simulink library "Solver_DS_SF"  (Simulink 7.1)
libraries: simulink x65
(part 1 of 2)
settings Model: Creator=Jin  LastModifiedBy=Jin

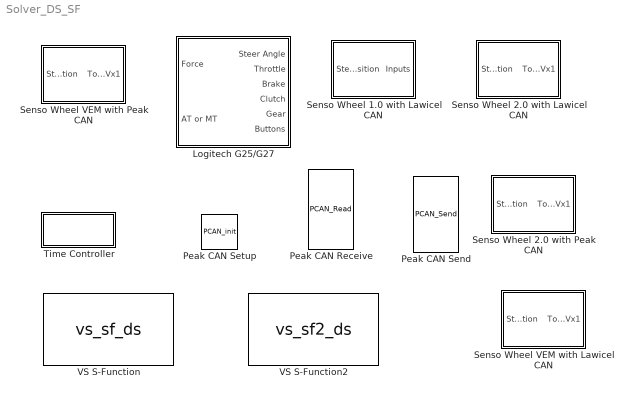
== system Solver_DS_SF ==
  Logitech G25/G27 : Subsystem
      mask Type: CarSim DS
      mask Description:
      | Logitech G25 Steering Wheel for CarSim/TruckSim Driving Simulator
      | 
      | Input 1: Force feedback
      | Input 2: AT mode (1), MT mode (-1)
      | 
      | Output 1: Steering Angle (-450deg - 450deg)
      | Output 2: Throttle position (0-1)
      | Output 3: Brake position (0-1)
      | Output 4: Clutch position (0-1)
      | Output 5: Gear shift
      |                 MT Mode:
      |                                 -1:  R
      |                               1-6: Gear 1-6
      |                 AT Mode:
      |                               button 1: Down shift
      |                               button 2: Upshift
      | Output 6: Other 14 buttons.
      mask Display: image(imread('G25.jpg'))
  Peak CAN Receive : S-Function  FunctionName=PCAN_Read  Parameters=id,TimeStep,nOut,bits_define  EnableBusSupport=off  mask{id=529, TimeStep=0.01, bits_define={[0:31],[32:47],[48:63]}, portnames={'Position','Speed','Motor Torque'}}
      mask prompts: id "CAN ID"; TimeStep "Sample time"; bits_define "Bit defination (cell array):"; portnames "Port name (cell array):"
      mask help: Peak-System USB CAN Receive.
      mask init:
      | %set_param(gcb, 'InitFcn', ['CAN_h=' adapter '_handle;']);
      | nOut=length(bits_define);
      | [bits_define]=formatbit(bits_define,portnames,1);
      | set_param(gcb, 'Parameters', ['id,TimeStep,nOut,bits_define']);
      mask Display: port_label('output',1,'Position ');port_label('output',2,'Speed ');port_label('output',3,'Motor Torque ');
  Peak CAN Send : S-Function  FunctionName=PCAN_Send  Parameters=id,len,TimeStep,nOut,bits_define  EnableBusSupport=off  mask{id=513, len=8, TimeStep=0.02, bits_define={[0:15],[16:31],[32:47],[48:63]}, portnames={'Torque Set Value','Friction','Damping','Spring Stiffness'}}
      mask prompts: id "CAN ID"; len "Data Length"; TimeStep "Sample time"; bits_define "Bit defination (cell array):"; portnames "Port name (cell array):"
      mask help: Peak-System USB CAN send
      mask init:
      | nOut=length(bits_define);
      | [bits_define]=formatbit(bits_define,portnames,0);
      | set_param(gcb, 'Parameters', ['id,len,TimeStep,nOut,bits_define']);
      mask StyleString: edit,popup(1|2|3|4|5|6|7|8),edit,edit,edit
      mask Display: port_label('input',1,' Torque Set Value');port_label('input',2,' Friction');port_label('input',3,' Damping');port_label('input',4,' Spring Stiffness');
  Peak CAN Setup : S-Function  Priority=1  FunctionName=PCAN_init  Parameters=CAN_MODE,szBitrate  EnableBusSupport=off  mask{CAN_MODE=Standard (11-bit), szBitrate=1000}
      mask prompts: CAN_MODE "CAN identifier range:"; szBitrate "Baud rate (kbps):"
      mask help: Peak-System USB CAN setup
      mask StyleString: popup(Standard (11-bit)|Extended (29-bit)),popup(1000|500|250|100|50|20|10|5)
      mask Display: image(imread('Peak_CAN.jpg'));
  Senso Wheel 1.0 with Lawicel CAN : Subsystem  Orientation=left  Priority=3
      mask Display: image(imread('SensoDrive.jpg'))
  Senso Wheel 2.0 with Lawicel CAN : Subsystem  Orientation=left  Priority=3
      mask Display: image(imread('SensoDrive.jpg'))
  Senso Wheel 2.0 with Peak CAN : Subsystem  Orientation=left  Priority=3
      mask Display: image(imread('SensoDrive.jpg'))
  Senso Wheel VEM with Lawicel CAN : Subsystem  Orientation=left  Priority=3
      mask Display: image(imread('SensoDrive.jpg'))
  Senso Wheel VEM with Peak CAN : Subsystem  Orientation=left  Priority=3  AncestorBlock=Solver_DS_SF/Senso Wheel 2.0 with Peak CAN
      mask Display: image(imread('SensoDrive.jpg'))
  Time Controller : Subsystem  AncestorBlock=Solver_SF/Time Controller  mask(CarSim DS){}
      mask help: This Real-Time control block enables the Simulink system running at real time mode.
      mask init:
      | TimeStep=str2num(get_param(gcs,'FixedStep'));
      mask Display: disp('RT Enable');
  VS S-Function : S-Function  Priority=1  FunctionName=vs_sf_ds  Parameters='simfile.sim'  EnableBusSupport=off  mask(Vehicle math model library){SIMFILE=simfile.sim}
      mask prompts: SIMFILE "Simfile name:"
      mask help:
      | The vehicle code on this S-Function determine which solver is used for vehicle type that is simulated.
      |
      | Simfile lists the names of the main files that will be read and written by the solver program.
      mask init:
      | set_param(gcb, 'Parameters', ['''',SIMFILE,'''']);
      mask Display: image(imread('car_ds.bmp'))
  VS S-Function2 : S-Function  Priority=1  FunctionName=vs_sf2_ds  Parameters='simfile.sim'  EnableBusSupport=off  mask(Vehicle math model library){SIMFILE=simfile.sim}
      mask prompts: SIMFILE "Simfile name:"
      mask help:
      | The vehicle code on this S-Function determine which solver is used for vehicle type that is simulated.
      |
      | Simfile lists the names of the main files that will be read and written by the solver program.
      mask init:
      | set_param(gcb, 'Parameters', ['''',SIMFILE,'''']);
      mask Display: image(imread('car_ds2.bmp'))

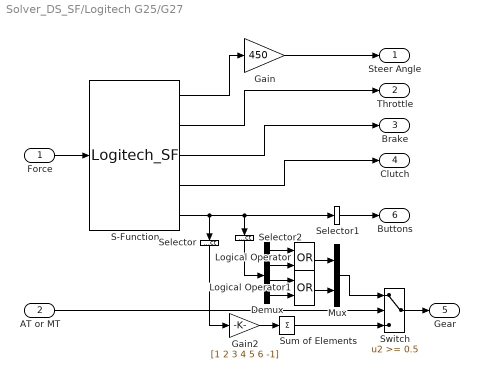
== system Solver_DS_SF/Logitech G25/G27 ==
  Force : Inport
  AT or MT : Inport  Port=2
  Demux : Demux
  Gain : Gain  Gain=450
  Gain2 : Gain  Gain=[1 2 3 4 5 6 -1]
  Logical Operator : Logic  Operator=OR  AllPortsSameDT=off  OutDataTypeStr=boolean  OutDataTypeMode=boolean
  Logical Operator1 : Logic  Operator=OR  AllPortsSameDT=off  OutDataTypeStr=boolean  OutDataTypeMode=boolean
  Mux : Mux  Inputs=2
  S-Function : S-Function  FunctionName=Logitech_SF  Parameters=19  EnableBusSupport=off
  Selector : Selector  Orientation=down  IndexOptions=Index vector (dialog)  Indices=[9 10 11 12 13 14 15]  OutputSizes=1
  Selector1 : Selector  IndexOptions=Index vector (dialog)  Indices=[1 2 3 4 5 6 7 8 16 17 18 19]  OutputSizes=1
  Selector2 : Selector  Orientation=down  IndexOptions=Index vector (dialog)  Indices=[9 6 10 5]  OutputSizes=1
  Sum of Elements : Sum  Inputs=+
  Switch : Switch  Threshold=0.5
  Steer Angle : Outport
  Throttle : Outport  Port=2
  Brake : Outport  Port=3
  Clutch : Outport  Port=4
  Gear : Outport  Port=5
  Buttons : Outport  Port=6
  wires:
  Mux/1 -> Switch/1
  Logical Operator1/1 -> Mux/2
  Logical Operator/1 -> Mux/1
  Demux/4 -> Logical Operator1/2
  Demux/3 -> Logical Operator1/1
  Demux/2 -> Logical Operator/2
  Demux/1 -> Logical Operator/1
  Selector2/1 -> Demux/1
  S-Function/1 -> Gain/1
  S-Function/2 -> Throttle/1
  Force/1 -> S-Function/1
  S-Function/3 -> Brake/1
  S-Function/4 -> Clutch/1
  S-Function/5 -> Selector2/1, Selector1/1, Selector/1
  Gain/1 -> Steer Angle/1
  Gain2/1 -> Sum of Elements/1
  Selector1/1 -> Buttons/1
  Selector/1 -> Gain2/1
  Sum of Elements/1 -> Switch/3
  AT or MT/1 -> Switch/2
  Switch/1 -> Gear/1

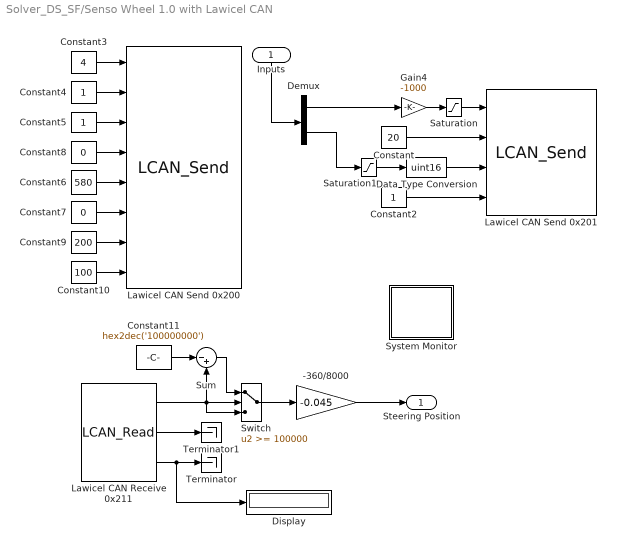
== system Solver_DS_SF/Senso Wheel 1.0 with Lawicel CAN ==
  Inputs : Inport  Orientation=down
  -360/8000 : Gain  Gain=-0.045  SaturateOnIntegerOverflow=on  OutDataTypeStr=Inherit: Same as input  ParamDataTypeStr=Inherit: Same as input
  Constant : Constant  Value=20  OutDataTypeStr=uint16  OutDataTypeMode=uint16
  Constant10 : Constant  Value=100  OutDataTypeStr=uint8  OutDataTypeMode=uint8
  Constant11 : Constant  Value=hex2dec('100000000')  VectorParams1D=off
  Constant2 : Constant  OutDataTypeStr=uint16  OutDataTypeMode=uint16
  Constant3 : Constant  Value=4  OutDataTypeStr=uint8  OutDataTypeMode=uint8
  Constant4 : Constant  OutDataTypeStr=uint8  OutDataTypeMode=uint8
  Constant5 : Constant  OutDataTypeStr=uint8  OutDataTypeMode=uint8
  Constant6 : Constant  Value=580  OutDataTypeStr=uint16  OutDataTypeMode=uint16
  Constant7 : Constant  Value=0  OutDataTypeStr=int16  OutDataTypeMode=int16
  Constant8 : Constant  Value=0  OutDataTypeStr=uint8  OutDataTypeMode=uint8
  Constant9 : Constant  Value=200  OutDataTypeStr=uint8  OutDataTypeMode=uint8
  Data Type Conversion : DataTypeConversion  OutDataTypeStr=uint16  OutDataTypeMode=uint16  RndMeth=Zero
  Demux : Demux  Outputs=2
  Display : Display
  Gain4 : Gain  Gain=-1000  SaturateOnIntegerOverflow=on  OutDataTypeStr=Inherit: Same as input  ParamDataTypeStr=Inherit: Same as input
  Lawicel CAN Receive 0x211 : S-Function  FunctionName=LCAN_Read  Parameters=1,CAN_MODE,id,TimeStep,nOut,bits_define  EnableBusSupport=off  mask{adapter=CAN1, CAN_MODE=Standard (11-bit), id=529, TimeStep=0.010, bits_define={[0:31],[32:47],[48:63]}, portnames={'Position','Speed','Motor Torque'}}
      mask prompts: adapter "CAN adapter"; CAN_MODE "CAN identifier range:"; id "CAN ID"; TimeStep "Sample time"; bits_define "Bit defination (cell array):"; portnames "Port name (cell array):"
      mask init:
      | nOut=length(bits_define);
      | [bits_define]=formatbit(bits_define,portnames,1);
      | set_param(gcb, 'Parameters', [adapter(4) ',CAN_MODE,id,TimeStep,nOut,bits_define']);
      mask StyleString: popup(CAN1|CAN2|CAN3|CAN4),popup(Standard (11-bit)|Extended (29-bit)),edit,edit,edit,edit
      mask Display: port_label('output',1,'Position ');port_label('output',2,'Speed ');port_label('output',3,'Motor Torque ');
  Lawicel CAN Send 0x200 : S-Function  FunctionName=LCAN_Send  Parameters=1,CAN_MODE,id,len,TimeStep,nOut,bits_define  EnableBusSupport=off  mask{adapter=CAN1, CAN_MODE=Standard (11-bit), id=512, len=8, TimeStep=0.025, bits_define={[0:3],[4:7],[8:11],[12:15],[16:31],[32:47],[48:55],[56:63]}, portnames={'Control Word','Operating Mode','Watch Dog','Position Limit','End Stop Position','Position Offset','Set Torque Limit','Peak Torque Limit'}}
      mask prompts: adapter "CAN adapter"; CAN_MODE "CAN identifier range:"; id "CAN ID"; len "Data Length"; TimeStep "Sample time"; bits_define "Bit defination (cell array):"; portnames "Port name (cell array):"
      mask init:
      | nOut=length(bits_define);
      | [bits_define]=formatbit(bits_define,portnames,0);
      | set_param(gcb, 'Parameters', [adapter(4) ',CAN_MODE,id,len,TimeStep,nOut,bits_define']);
      mask StyleString: popup(CAN1|CAN2|CAN3|CAN4),popup(Standard (11-bit)|Extended (29-bit)),edit,popup(1|2|3|4|5|6|7|8),edit,edit,edit
      mask Display: port_label('input',1,' Control Word');port_label('input',2,' Operating Mode');port_label('input',3,' Watch Dog');port_label('input',4,' Position Limit');port_label('input',5,' End Stop Position');port_label('input',6,' Position Offset');port_label('input',7,' Set Torque Limit');port_label('input',8,' Peak Torque Limit');
  Lawicel CAN Send 0x201 : S-Function  FunctionName=LCAN_Send  Parameters=1,CAN_MODE,id,len,TimeStep,nOut,bits_define  EnableBusSupport=off  mask{adapter=CAN1, CAN_MODE=Standard (11-bit), id=513, len=8, TimeStep=0.02, bits_define={[0:15],[16:31],[32:47],[48:63]}, portnames={'Torque Set Value','Friction','Damping','Spring Stiffness'}}
      mask prompts: adapter "CAN adapter"; CAN_MODE "CAN identifier range:"; id "CAN ID"; len "Data Length"; TimeStep "Sample time"; bits_define "Bit defination (cell array):"; portnames "Port name (cell array):"
      mask init:
      | nOut=length(bits_define);
      | [bits_define]=formatbit(bits_define,portnames,0);
      | set_param(gcb, 'Parameters', [adapter(4) ',CAN_MODE,id,len,TimeStep,nOut,bits_define']);
      mask StyleString: popup(CAN1|CAN2|CAN3|CAN4),popup(Standard (11-bit)|Extended (29-bit)),edit,popup(1|2|3|4|5|6|7|8),edit,edit,edit
      mask Display: port_label('input',1,' Torque Set Value');port_label('input',2,' Friction');port_label('input',3,' Damping');port_label('input',4,' Spring Stiffness');
  Saturation : Saturate  UpperLimit=14500  LowerLimit=-14500
  Saturation1 : Saturate  UpperLimit=200  LowerLimit=40
  Sum : Sum  Inputs=|-+  SaturateOnIntegerOverflow=on
  Switch : Switch  Threshold=100000  SaturateOnIntegerOverflow=on
  System Monitor : Subsystem
  Terminator : Terminator
  Terminator1 : Terminator
  Steering Position : Outport
  wires:
  Constant/1 -> Lawicel CAN Send 0x201/2
  Constant2/1 -> Lawicel CAN Send 0x201/4
  Constant3/1 -> Lawicel CAN Send 0x200/1
  Constant4/1 -> Lawicel CAN Send 0x200/2
  Constant5/1 -> Lawicel CAN Send 0x200/3
  Constant8/1 -> Lawicel CAN Send 0x200/4
  Constant6/1 -> Lawicel CAN Send 0x200/5
  Constant7/1 -> Lawicel CAN Send 0x200/6
  Constant9/1 -> Lawicel CAN Send 0x200/7
  Constant10/1 -> Lawicel CAN Send 0x200/8
  Lawicel CAN Receive 0x211/2 -> Terminator1/1
  Lawicel CAN Receive 0x211/3 -> Terminator/1, Display/1
  Lawicel CAN Receive 0x211/1 -> Sum/2, Switch/2, Switch/3
  -360/8000/1 -> Steering Position/1
  Gain4/1 -> Saturation/1
  Saturation/1 -> Lawicel CAN Send 0x201/1
  Constant11/1 -> Sum/1
  Sum/1 -> Switch/1
  Switch/1 -> -360/8000/1
  Inputs/1 -> Demux/1
  Demux/1 -> Gain4/1
  Demux/2 -> Saturation1/1
  Saturation1/1 -> Data Type Conversion/1
  Data Type Conversion/1 -> Lawicel CAN Send 0x201/3

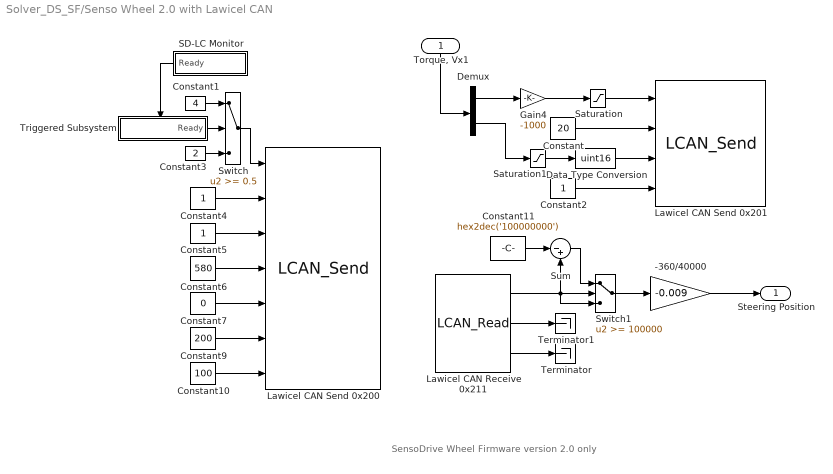
== system Solver_DS_SF/Senso Wheel 2.0 with Lawicel CAN ==
  note: SensoDrive Wheel Firmware version 2.0 only
  "Torque, Vx1" : Inport  Orientation=down
  -360/40000 : Gain  Gain=-0.009  SaturateOnIntegerOverflow=on  OutDataTypeStr=Inherit: Same as input  ParamDataTypeStr=Inherit: Same as input
  Constant : Constant  Value=20  OutDataTypeStr=uint16  OutDataTypeMode=uint16
  Constant1 : Constant  Value=4  OutDataTypeStr=uint8  OutDataTypeMode=uint8
  Constant10 : Constant  Value=100  OutDataTypeStr=uint8  OutDataTypeMode=uint8
  Constant11 : Constant  Value=hex2dec('100000000')  VectorParams1D=off
  Constant2 : Constant  OutDataTypeStr=uint16  OutDataTypeMode=uint16
  Constant3 : Constant  Value=2  OutDataTypeStr=uint8  OutDataTypeMode=uint8
  Constant4 : Constant  OutDataTypeStr=uint8  OutDataTypeMode=uint8
  Constant5 : Constant  OutDataTypeStr=uint8  OutDataTypeMode=uint8
  Constant6 : Constant  Value=580  OutDataTypeStr=uint16  OutDataTypeMode=uint16
  Constant7 : Constant  Value=0  OutDataTypeStr=int16  OutDataTypeMode=int16
  Constant9 : Constant  Value=200  OutDataTypeStr=uint8  OutDataTypeMode=uint8
  Data Type Conversion : DataTypeConversion  OutDataTypeStr=uint16  OutDataTypeMode=uint16  RndMeth=Zero
  Demux : Demux  Outputs=2
  Gain4 : Gain  Gain=-1000  SaturateOnIntegerOverflow=on  OutDataTypeStr=Inherit: Same as input  ParamDataTypeStr=Inherit: Same as input
  Lawicel CAN Receive 0x211 : S-Function  FunctionName=LCAN_Read  Parameters=1,CAN_MODE,id,TimeStep,nOut,bits_define  EnableBusSupport=off  mask{adapter=CAN1, CAN_MODE=Standard (11-bit), id=529, TimeStep=0.010, bits_define={[0:31],[32:47],[48:63]}, portnames={'Position','Speed','Motor Torque'}}
      mask prompts: adapter "CAN adapter"; CAN_MODE "CAN identifier range:"; id "CAN ID"; TimeStep "Sample time"; bits_define "Bit defination (cell array):"; portnames "Port name (cell array):"
      mask init:
      | nOut=length(bits_define);
      | [bits_define]=formatbit(bits_define,portnames,1);
      | set_param(gcb, 'Parameters', [adapter(4) ',CAN_MODE,id,TimeStep,nOut,bits_define']);
      mask StyleString: popup(CAN1|CAN2|CAN3|CAN4),popup(Standard (11-bit)|Extended (29-bit)),edit,edit,edit,edit
      mask Display: port_label('output',1,'Position ');port_label('output',2,'Speed ');port_label('output',3,'Motor Torque ');
  Lawicel CAN Send 0x200 : S-Function  Priority=3  FunctionName=LCAN_Send  Parameters=1,CAN_MODE,id,len,TimeStep,nOut,bits_define  EnableBusSupport=off  mask{adapter=CAN1, CAN_MODE=Standard (11-bit), id=512, len=8, TimeStep=0.025, bits_define={[0:3],[4:7],[8:15],[16:31],[32:47],[48:55],[56:63]}, portnames={'Control Word','Operating Mode','Aux. Functions','End Stop Position','Position Offset','Set Torque Limit','Peak Torque Limit'}}
      mask prompts: adapter "CAN adapter"; CAN_MODE "CAN identifier range:"; id "CAN ID"; len "Data Length"; TimeStep "Sample time"; bits_define "Bit defination (cell array):"; portnames "Port name (cell array):"
      mask init:
      | nOut=length(bits_define);
      | [bits_define]=formatbit(bits_define,portnames,0);
      | set_param(gcb, 'Parameters', [adapter(4) ',CAN_MODE,id,len,TimeStep,nOut,bits_define']);
      mask StyleString: popup(CAN1|CAN2|CAN3|CAN4),popup(Standard (11-bit)|Extended (29-bit)),edit,popup(1|2|3|4|5|6|7|8),edit,edit,edit
      mask Display: port_label('input',1,' Control Word');port_label('input',2,' Operating Mode');port_label('input',3,' Aux. Functions');port_label('input',4,' End Stop Position');port_label('input',5,' Position Offset');port_label('input',6,' Set Torque Limit');port_label('input',7,' Peak Torque Limit');
  Lawicel CAN Send 0x201 : S-Function  FunctionName=LCAN_Send  Parameters=1,CAN_MODE,id,len,TimeStep,nOut,bits_define  EnableBusSupport=off  mask{adapter=CAN1, CAN_MODE=Standard (11-bit), id=513, len=8, TimeStep=0.02, bits_define={[0:15],[16:31],[32:47],[48:63]}, portnames={'Torque Set Value','Friction','Damping','Spring Stiffness'}}
      mask prompts: adapter "CAN adapter"; CAN_MODE "CAN identifier range:"; id "CAN ID"; len "Data Length"; TimeStep "Sample time"; bits_define "Bit defination (cell array):"; portnames "Port name (cell array):"
      mask init:
      | nOut=length(bits_define);
      | [bits_define]=formatbit(bits_define,portnames,0);
      | set_param(gcb, 'Parameters', [adapter(4) ',CAN_MODE,id,len,TimeStep,nOut,bits_define']);
      mask StyleString: popup(CAN1|CAN2|CAN3|CAN4),popup(Standard (11-bit)|Extended (29-bit)),edit,popup(1|2|3|4|5|6|7|8),edit,edit,edit
      mask Display: port_label('input',1,' Torque Set Value');port_label('input',2,' Friction');port_label('input',3,' Damping');port_label('input',4,' Spring Stiffness');
  SD-LC Monitor : Subsystem  Orientation=left  Priority=4
  Saturation : Saturate  UpperLimit=14500  LowerLimit=-14500
  Saturation1 : Saturate  UpperLimit=200  LowerLimit=40
  Sum : Sum  Inputs=|-+  SaturateOnIntegerOverflow=on
  Switch : Switch  Threshold=0.5  SaturateOnIntegerOverflow=on
  Switch1 : Switch  Threshold=100000  SaturateOnIntegerOverflow=on
  Terminator : Terminator
  Terminator1 : Terminator
  Triggered Subsystem : Subsystem  TreatAsAtomicUnit=on
  Steering Position : Outport
  wires:
  Switch1/1 -> -360/40000/1
  Sum/1 -> Switch1/1
  Constant11/1 -> Sum/1
  -360/40000/1 -> Steering Position/1
  Lawicel CAN Receive 0x211/1 -> Sum/2, Switch1/2, Switch1/3
  Lawicel CAN Receive 0x211/3 -> Terminator/1
  Lawicel CAN Receive 0x211/2 -> Terminator1/1
  Data Type Conversion/1 -> Lawicel CAN Send 0x201/3
  Saturation1/1 -> Data Type Conversion/1
  Demux/2 -> Saturation1/1
  Demux/1 -> Gain4/1
  "Torque, Vx1"/1 -> Demux/1
  Saturation/1 -> Lawicel CAN Send 0x201/1
  Gain4/1 -> Saturation/1
  Constant2/1 -> Lawicel CAN Send 0x201/4
  Constant/1 -> Lawicel CAN Send 0x201/2
  Triggered Subsystem/1(Ready) -> Switch/2
  Constant1/1 -> Switch/1
  Constant3/1 -> Switch/3
  Switch/1 -> Lawicel CAN Send 0x200/1
  SD-LC Monitor/1(Ready) -> Triggered Subsystem/Trigger
  Constant10/1 -> Lawicel CAN Send 0x200/7
  Constant9/1 -> Lawicel CAN Send 0x200/6
  Constant7/1 -> Lawicel CAN Send 0x200/5
  Constant6/1 -> Lawicel CAN Send 0x200/4
  Constant5/1 -> Lawicel CAN Send 0x200/3
  Constant4/1 -> Lawicel CAN Send 0x200/2

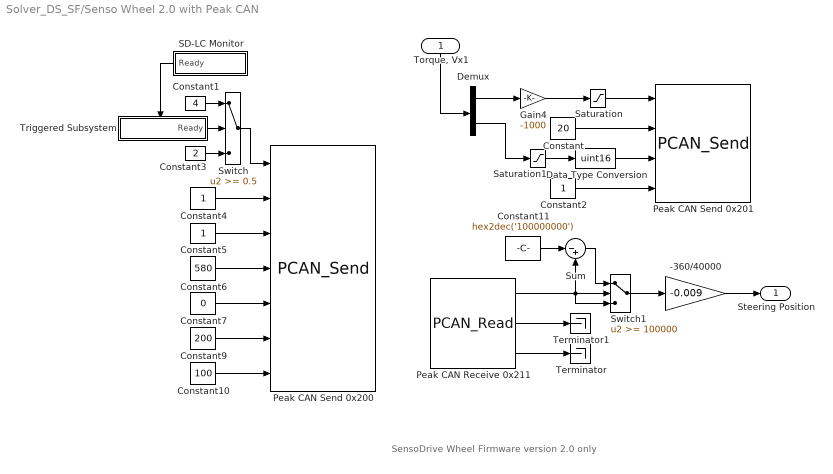
== system Solver_DS_SF/Senso Wheel 2.0 with Peak CAN ==
  note: SensoDrive Wheel Firmware version 2.0 only
  "Torque, Vx1" : Inport  Orientation=down
  -360/40000 : Gain  Gain=-0.009  SaturateOnIntegerOverflow=on  OutDataTypeStr=Inherit: Same as input  ParamDataTypeStr=Inherit: Same as input
  Constant : Constant  Value=20  OutDataTypeStr=uint16  OutDataTypeMode=uint16
  Constant1 : Constant  Value=4  OutDataTypeStr=uint8  OutDataTypeMode=uint8
  Constant10 : Constant  Value=100  OutDataTypeStr=uint8  OutDataTypeMode=uint8
  Constant11 : Constant  Value=hex2dec('100000000')  VectorParams1D=off
  Constant2 : Constant  OutDataTypeStr=uint16  OutDataTypeMode=uint16
  Constant3 : Constant  Value=2  OutDataTypeStr=uint8  OutDataTypeMode=uint8
  Constant4 : Constant  OutDataTypeStr=uint8  OutDataTypeMode=uint8
  Constant5 : Constant  OutDataTypeStr=uint8  OutDataTypeMode=uint8
  Constant6 : Constant  Value=580  OutDataTypeStr=uint16  OutDataTypeMode=uint16
  Constant7 : Constant  Value=0  OutDataTypeStr=int16  OutDataTypeMode=int16
  Constant9 : Constant  Value=200  OutDataTypeStr=uint8  OutDataTypeMode=uint8
  Data Type Conversion : DataTypeConversion  OutDataTypeStr=uint16  OutDataTypeMode=uint16  RndMeth=Zero
  Demux : Demux  Outputs=2
  Gain4 : Gain  Gain=-1000  SaturateOnIntegerOverflow=on  OutDataTypeStr=Inherit: Same as input  ParamDataTypeStr=Inherit: Same as input
  Peak CAN Receive 0x211 : S-Function  AncestorBlock=Solver_SF/Lawicel CAN Receive  FunctionName=PCAN_Read  Parameters=id,TimeStep,nOut,bits_define  EnableBusSupport=off  mask(CarSim DS){id=529, TimeStep=0.01, bits_define={[0:31],[32:47],[48:63]}, portnames={'Position','Speed','Motor Torque'}}
      mask prompts: id "CAN ID"; TimeStep "Sample time"; bits_define "Bit defination (cell array):"; portnames "Port name (cell array):"
      mask help: Lawicel CAN Receive.
      mask init:
      | nOut=length(bits_define);
      | [bits_define]=formatbit(bits_define,portnames,1);
      | set_param(gcb, 'Parameters', ['id,TimeStep,nOut,bits_define']);
      mask Display: port_label('output',1,'Position ');port_label('output',2,'Speed ');port_label('output',3,'Motor Torque ');
  Peak CAN Send 0x200 : S-Function  AncestorBlock=Solver_SF/Peak CAN Send  FunctionName=PCAN_Send  Parameters=id,len,TimeStep,nOut,bits_define  EnableBusSupport=off  mask{id=512, len=8, TimeStep=0.025, bits_define={[0:3],[4:7],[8:15],[16:31],[32:47],[48:55],[56:63]}, portnames={'Control Word','Operating Mode','Aux. Functions','End Stop Position','Position Offset','Set Torque Limit','Peak Torque Limit'}}
      mask prompts: id "CAN ID"; len "Data Length"; TimeStep "Sample time"; bits_define "Bit defination (cell array):"; portnames "Port name (cell array):"
      mask help: Peak-System USB CAN send
      mask init:
      | nOut=length(bits_define);
      | [bits_define]=formatbit(bits_define,portnames,0);
      | set_param(gcb, 'Parameters', ['id,len,TimeStep,nOut,bits_define']);
      mask StyleString: edit,popup(1|2|3|4|5|6|7|8),edit,edit,edit
      mask Display: port_label('input',1,' Control Word');port_label('input',2,' Operating Mode');port_label('input',3,' Aux. Functions');port_label('input',4,' End Stop Position');port_label('input',5,' Position Offset');port_label('input',6,' Set Torque Limit');port_label('input',7,' Peak Torque Limit');
  Peak CAN Send 0x201 : S-Function  AncestorBlock=Solver_SF/Peak CAN Send  FunctionName=PCAN_Send  Parameters=id,len,TimeStep,nOut,bits_define  EnableBusSupport=off  mask{id=513, len=8, TimeStep=0.02, bits_define={[0:15],[16:31],[32:47],[48:63]}, portnames={'Torque Set Value','Friction','Damping','Spring Stiffness'}}
      mask prompts: id "CAN ID"; len "Data Length"; TimeStep "Sample time"; bits_define "Bit defination (cell array):"; portnames "Port name (cell array):"
      mask help: Peak-System USB CAN send
      mask init:
      | nOut=length(bits_define);
      | [bits_define]=formatbit(bits_define,portnames,0);
      | set_param(gcb, 'Parameters', ['id,len,TimeStep,nOut,bits_define']);
      mask StyleString: edit,popup(1|2|3|4|5|6|7|8),edit,edit,edit
      mask Display: port_label('input',1,' Torque Set Value');port_label('input',2,' Friction');port_label('input',3,' Damping');port_label('input',4,' Spring Stiffness');
  SD-LC Monitor : Subsystem  Orientation=left  Priority=4
  Saturation : Saturate  UpperLimit=14500  LowerLimit=-14500
  Saturation1 : Saturate  UpperLimit=200  LowerLimit=40
  Sum : Sum  Inputs=|-+  SaturateOnIntegerOverflow=on
  Switch : Switch  Threshold=0.5  SaturateOnIntegerOverflow=on
  Switch1 : Switch  Threshold=100000  SaturateOnIntegerOverflow=on
  Terminator : Terminator
  Terminator1 : Terminator
  Triggered Subsystem : Subsystem  TreatAsAtomicUnit=on
  Steering Position : Outport
  wires:
  Switch1/1 -> -360/40000/1
  Sum/1 -> Switch1/1
  Constant11/1 -> Sum/1
  -360/40000/1 -> Steering Position/1
  Peak CAN Receive 0x211/1 -> Sum/2, Switch1/2, Switch1/3
  Peak CAN Receive 0x211/3 -> Terminator/1
  Peak CAN Receive 0x211/2 -> Terminator1/1
  Data Type Conversion/1 -> Peak CAN Send 0x201/3
  Saturation1/1 -> Data Type Conversion/1
  Demux/2 -> Saturation1/1
  Demux/1 -> Gain4/1
  "Torque, Vx1"/1 -> Demux/1
  Saturation/1 -> Peak CAN Send 0x201/1
  Gain4/1 -> Saturation/1
  Constant2/1 -> Peak CAN Send 0x201/4
  Constant/1 -> Peak CAN Send 0x201/2
  Triggered Subsystem/1(Ready) -> Switch/2
  Constant1/1 -> Switch/1
  Constant3/1 -> Switch/3
  Switch/1 -> Peak CAN Send 0x200/1
  SD-LC Monitor/1(Ready) -> Triggered Subsystem/Trigger
  Constant10/1 -> Peak CAN Send 0x200/7
  Constant9/1 -> Peak CAN Send 0x200/6
  Constant7/1 -> Peak CAN Send 0x200/5
  Constant6/1 -> Peak CAN Send 0x200/4
  Constant5/1 -> Peak CAN Send 0x200/3
  Constant4/1 -> Peak CAN Send 0x200/2

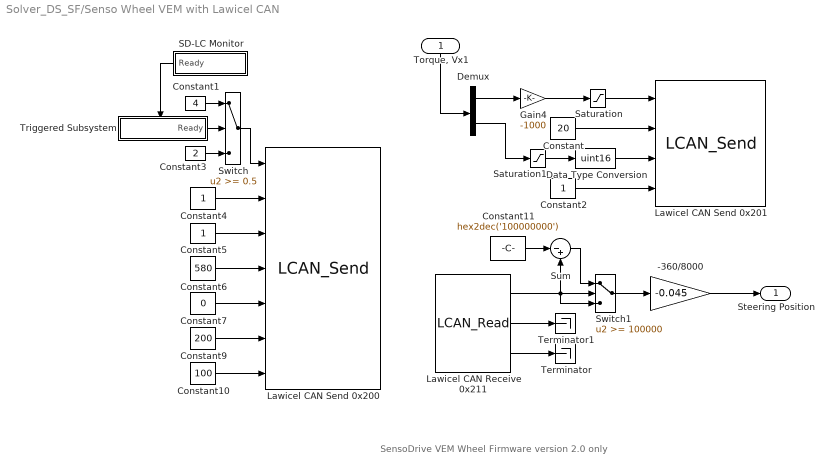
== system Solver_DS_SF/Senso Wheel VEM with Lawicel CAN ==
  note: SensoDrive VEM Wheel Firmware version 2.0 only
  "Torque, Vx1" : Inport  Orientation=down
  -360/8000 : Gain  Gain=-0.045  SaturateOnIntegerOverflow=on  OutDataTypeStr=Inherit: Same as input  ParamDataTypeStr=Inherit: Same as input
  Constant : Constant  Value=20  OutDataTypeStr=uint16  OutDataTypeMode=uint16
  Constant1 : Constant  Value=4  OutDataTypeStr=uint8  OutDataTypeMode=uint8
  Constant10 : Constant  Value=100  OutDataTypeStr=uint8  OutDataTypeMode=uint8
  Constant11 : Constant  Value=hex2dec('100000000')  VectorParams1D=off
  Constant2 : Constant  OutDataTypeStr=uint16  OutDataTypeMode=uint16
  Constant3 : Constant  Value=2  OutDataTypeStr=uint8  OutDataTypeMode=uint8
  Constant4 : Constant  OutDataTypeStr=uint8  OutDataTypeMode=uint8
  Constant5 : Constant  OutDataTypeStr=uint8  OutDataTypeMode=uint8
  Constant6 : Constant  Value=580  OutDataTypeStr=uint16  OutDataTypeMode=uint16
  Constant7 : Constant  Value=0  OutDataTypeStr=int16  OutDataTypeMode=int16
  Constant9 : Constant  Value=200  OutDataTypeStr=uint8  OutDataTypeMode=uint8
  Data Type Conversion : DataTypeConversion  OutDataTypeStr=uint16  OutDataTypeMode=uint16  RndMeth=Zero
  Demux : Demux  Outputs=2
  Gain4 : Gain  Gain=-1000  SaturateOnIntegerOverflow=on  OutDataTypeStr=Inherit: Same as input  ParamDataTypeStr=Inherit: Same as input
  Lawicel CAN Receive 0x211 : S-Function  FunctionName=LCAN_Read  Parameters=1,CAN_MODE,id,TimeStep,nOut,bits_define  EnableBusSupport=off  mask{adapter=CAN1, CAN_MODE=Standard (11-bit), id=529, TimeStep=0.010, bits_define={[0:31],[32:47],[48:63]}, portnames={'Position','Speed','Motor Torque'}}
      mask prompts: adapter "CAN adapter"; CAN_MODE "CAN identifier range:"; id "CAN ID"; TimeStep "Sample time"; bits_define "Bit defination (cell array):"; portnames "Port name (cell array):"
      mask init:
      | nOut=length(bits_define);
      | [bits_define]=formatbit(bits_define,portnames,1);
      | set_param(gcb, 'Parameters', [adapter(4) ',CAN_MODE,id,TimeStep,nOut,bits_define']);
      mask StyleString: popup(CAN1|CAN2|CAN3|CAN4),popup(Standard (11-bit)|Extended (29-bit)),edit,edit,edit,edit
      mask Display: port_label('output',1,'Position ');port_label('output',2,'Speed ');port_label('output',3,'Motor Torque ');
  Lawicel CAN Send 0x200 : S-Function  Priority=3  FunctionName=LCAN_Send  Parameters=1,CAN_MODE,id,len,TimeStep,nOut,bits_define  EnableBusSupport=off  mask{adapter=CAN1, CAN_MODE=Standard (11-bit), id=512, len=8, TimeStep=0.025, bits_define={[0:3],[4:7],[8:15],[16:31],[32:47],[48:55],[56:63]}, portnames={'Control Word','Operating Mode','Aux. Functions','End Stop Position','Position Offset','Set Torque Limit','Peak Torque Limit'}}
      mask prompts: adapter "CAN adapter"; CAN_MODE "CAN identifier range:"; id "CAN ID"; len "Data Length"; TimeStep "Sample time"; bits_define "Bit defination (cell array):"; portnames "Port name (cell array):"
      mask init:
      | nOut=length(bits_define);
      | [bits_define]=formatbit(bits_define,portnames,0);
      | set_param(gcb, 'Parameters', [adapter(4) ',CAN_MODE,id,len,TimeStep,nOut,bits_define']);
      mask StyleString: popup(CAN1|CAN2|CAN3|CAN4),popup(Standard (11-bit)|Extended (29-bit)),edit,popup(1|2|3|4|5|6|7|8),edit,edit,edit
      mask Display: port_label('input',1,' Control Word');port_label('input',2,' Operating Mode');port_label('input',3,' Aux. Functions');port_label('input',4,' End Stop Position');port_label('input',5,' Position Offset');port_label('input',6,' Set Torque Limit');port_label('input',7,' Peak Torque Limit');
  Lawicel CAN Send 0x201 : S-Function  FunctionName=LCAN_Send  Parameters=1,CAN_MODE,id,len,TimeStep,nOut,bits_define  EnableBusSupport=off  mask{adapter=CAN1, CAN_MODE=Standard (11-bit), id=513, len=8, TimeStep=0.02, bits_define={[0:15],[16:31],[32:47],[48:63]}, portnames={'Torque Set Value','Friction','Damping','Spring Stiffness'}}
      mask prompts: adapter "CAN adapter"; CAN_MODE "CAN identifier range:"; id "CAN ID"; len "Data Length"; TimeStep "Sample time"; bits_define "Bit defination (cell array):"; portnames "Port name (cell array):"
      mask init:
      | nOut=length(bits_define);
      | [bits_define]=formatbit(bits_define,portnames,0);
      | set_param(gcb, 'Parameters', [adapter(4) ',CAN_MODE,id,len,TimeStep,nOut,bits_define']);
      mask StyleString: popup(CAN1|CAN2|CAN3|CAN4),popup(Standard (11-bit)|Extended (29-bit)),edit,popup(1|2|3|4|5|6|7|8),edit,edit,edit
      mask Display: port_label('input',1,' Torque Set Value');port_label('input',2,' Friction');port_label('input',3,' Damping');port_label('input',4,' Spring Stiffness');
  SD-LC Monitor : Subsystem  Orientation=left  Priority=4
  Saturation : Saturate  UpperLimit=14500  LowerLimit=-14500
  Saturation1 : Saturate  UpperLimit=200  LowerLimit=40
  Sum : Sum  Inputs=|-+  SaturateOnIntegerOverflow=on
  Switch : Switch  Threshold=0.5  SaturateOnIntegerOverflow=on
  Switch1 : Switch  Threshold=100000  SaturateOnIntegerOverflow=on
  Terminator : Terminator
  Terminator1 : Terminator
  Triggered Subsystem : Subsystem  TreatAsAtomicUnit=on
  Steering Position : Outport
  wires:
  Switch1/1 -> -360/8000/1
  Sum/1 -> Switch1/1
  Constant11/1 -> Sum/1
  -360/8000/1 -> Steering Position/1
  Lawicel CAN Receive 0x211/1 -> Sum/2, Switch1/2, Switch1/3
  Lawicel CAN Receive 0x211/3 -> Terminator/1
  Lawicel CAN Receive 0x211/2 -> Terminator1/1
  Data Type Conversion/1 -> Lawicel CAN Send 0x201/3
  Saturation1/1 -> Data Type Conversion/1
  Demux/2 -> Saturation1/1
  Demux/1 -> Gain4/1
  "Torque, Vx1"/1 -> Demux/1
  Saturation/1 -> Lawicel CAN Send 0x201/1
  Gain4/1 -> Saturation/1
  Constant2/1 -> Lawicel CAN Send 0x201/4
  Constant/1 -> Lawicel CAN Send 0x201/2
  Triggered Subsystem/1(Ready) -> Switch/2
  Constant1/1 -> Switch/1
  Constant3/1 -> Switch/3
  Switch/1 -> Lawicel CAN Send 0x200/1
  SD-LC Monitor/1(Ready) -> Triggered Subsystem/Trigger
  Constant10/1 -> Lawicel CAN Send 0x200/7
  Constant9/1 -> Lawicel CAN Send 0x200/6
  Constant7/1 -> Lawicel CAN Send 0x200/5
  Constant6/1 -> Lawicel CAN Send 0x200/4
  Constant5/1 -> Lawicel CAN Send 0x200/3
  Constant4/1 -> Lawicel CAN Send 0x200/2

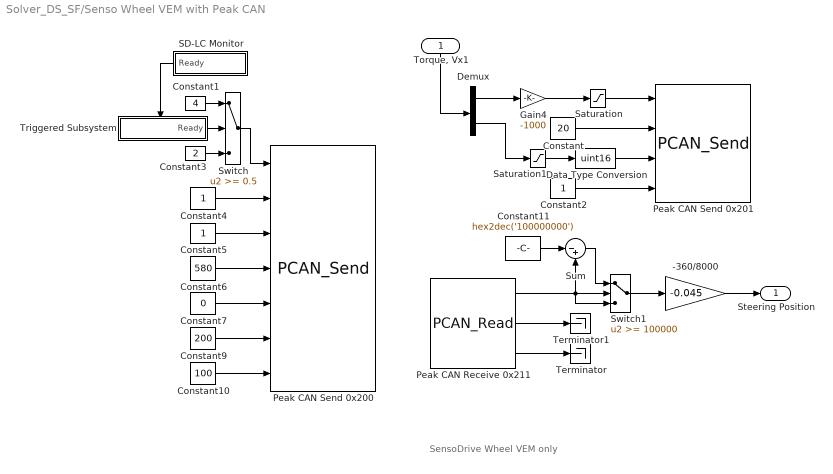
== system Solver_DS_SF/Senso Wheel VEM with Peak CAN ==
  note: SensoDrive Wheel VEM only
  "Torque, Vx1" : Inport  Orientation=down
  -360/8000 : Gain  Gain=-0.045  SaturateOnIntegerOverflow=on  OutDataTypeStr=Inherit: Same as input  ParamDataTypeStr=Inherit: Same as input
  Constant : Constant  Value=20  OutDataTypeStr=uint16  OutDataTypeMode=uint16
  Constant1 : Constant  Value=4  OutDataTypeStr=uint8  OutDataTypeMode=uint8
  Constant10 : Constant  Value=100  OutDataTypeStr=uint8  OutDataTypeMode=uint8
  Constant11 : Constant  Value=hex2dec('100000000')  VectorParams1D=off
  Constant2 : Constant  OutDataTypeStr=boolean  OutDataTypeMode=boolean
  Constant3 : Constant  Value=2  OutDataTypeStr=boolean  OutDataTypeMode=boolean
  Constant4 : Constant  OutDataTypeStr=uint8  OutDataTypeMode=uint8
  Constant5 : Constant  OutDataTypeStr=uint8  OutDataTypeMode=uint8
  Constant6 : Constant  Value=580  OutDataTypeStr=boolean  OutDataTypeMode=boolean
  Constant7 : Constant  Value=0  OutDataTypeStr=boolean  OutDataTypeMode=boolean
  Constant9 : Constant  Value=200  OutDataTypeStr=uint8  OutDataTypeMode=uint8
  Data Type Conversion : DataTypeConversion  OutDataTypeStr=uint16  OutDataTypeMode=uint16  RndMeth=Zero
  Demux : Demux  Outputs=2
  Gain4 : Gain  Gain=-1000  SaturateOnIntegerOverflow=on  OutDataTypeStr=Inherit: Same as input  ParamDataTypeStr=Inherit: Same as input
  Peak CAN Receive 0x211 : S-Function  AncestorBlock=Solver_SF/Lawicel CAN Receive  FunctionName=PCAN_Read  Parameters=id,TimeStep,nOut,bits_define  EnableBusSupport=off  mask(CarSim DS){id=529, TimeStep=0.01, bits_define={[0:31],[32:47],[48:63]}, portnames={'Position','Speed','Motor Torque'}}
      mask prompts: id "CAN ID"; TimeStep "Sample time"; bits_define "Bit defination (cell array):"; portnames "Port name (cell array):"
      mask help: Lawicel CAN Receive.
      mask init:
      | nOut=length(bits_define);
      | [bits_define]=formatbit(bits_define,portnames,1);
      | set_param(gcb, 'Parameters', ['id,TimeStep,nOut,bits_define']);
      mask Display: port_label('output',1,'Position ');port_label('output',2,'Speed ');port_label('output',3,'Motor Torque ');
  Peak CAN Send 0x200 : S-Function  AncestorBlock=Solver_SF/Peak CAN Send  FunctionName=PCAN_Send  Parameters=id,len,TimeStep,nOut,bits_define  EnableBusSupport=off  mask{id=512, len=8, TimeStep=0.025, bits_define={[0:3],[4:7],[8:15],[16:31],[32:47],[48:55],[56:63]}, portnames={'Control Word','Operating Mode','Aux. Functions','End Stop Position','Position Offset','Set Torque Limit','Peak Torque Limit'}}
      mask prompts: id "CAN ID"; len "Data Length"; TimeStep "Sample time"; bits_define "Bit defination (cell array):"; portnames "Port name (cell array):"
      mask help: Peak-System USB CAN send
      mask init:
      | nOut=length(bits_define);
      | [bits_define]=formatbit(bits_define,portnames,0);
      | set_param(gcb, 'Parameters', ['id,len,TimeStep,nOut,bits_define']);
      mask StyleString: edit,popup(1|2|3|4|5|6|7|8),edit,edit,edit
      mask Display: port_label('input',1,' Control Word');port_label('input',2,' Operating Mode');port_label('input',3,' Aux. Functions');port_label('input',4,' End Stop Position');port_label('input',5,' Position Offset');port_label('input',6,' Set Torque Limit');port_label('input',7,' Peak Torque Limit');
  Peak CAN Send 0x201 : S-Function  AncestorBlock=Solver_SF/Peak CAN Send  FunctionName=PCAN_Send  Parameters=id,len,TimeStep,nOut,bits_define  EnableBusSupport=off  mask{id=513, len=8, TimeStep=0.02, bits_define={[0:15],[16:31],[32:47],[48:63]}, portnames={'Torque Set Value','Friction','Damping','Spring Stiffness'}}
      mask prompts: id "CAN ID"; len "Data Length"; TimeStep "Sample time"; bits_define "Bit defination (cell array):"; portnames "Port name (cell array):"
      mask help: Peak-System USB CAN send
      mask init:
      | nOut=length(bits_define);
      | [bits_define]=formatbit(bits_define,portnames,0);
      | set_param(gcb, 'Parameters', ['id,len,TimeStep,nOut,bits_define']);
      mask StyleString: edit,popup(1|2|3|4|5|6|7|8),edit,edit,edit
      mask Display: port_label('input',1,' Torque Set Value');port_label('input',2,' Friction');port_label('input',3,' Damping');port_label('input',4,' Spring Stiffness');
  SD-LC Monitor : Subsystem  Orientation=left  Priority=4
  Saturation : Saturate  UpperLimit=14500  LowerLimit=-14500
  Saturation1 : Saturate  UpperLimit=200  LowerLimit=40
  Sum : Sum  Inputs=|-+  SaturateOnIntegerOverflow=on
  Switch : Switch  Threshold=0.5  SaturateOnIntegerOverflow=on
  Switch1 : Switch  Threshold=100000  SaturateOnIntegerOverflow=on
  Terminator : Terminator
  Terminator1 : Terminator
  Triggered Subsystem : Subsystem  TreatAsAtomicUnit=on
  Steering Position : Outport
  wires:
  Switch1/1 -> -360/8000/1
  Sum/1 -> Switch1/1
  Constant11/1 -> Sum/1
  -360/8000/1 -> Steering Position/1
  Peak CAN Receive 0x211/1 -> Sum/2, Switch1/2, Switch1/3
  Peak CAN Receive 0x211/3 -> Terminator/1
  Peak CAN Receive 0x211/2 -> Terminator1/1
  Data Type Conversion/1 -> Peak CAN Send 0x201/3
  Saturation1/1 -> Data Type Conversion/1
  Demux/2 -> Saturation1/1
  Demux/1 -> Gain4/1
  "Torque, Vx1"/1 -> Demux/1
  Saturation/1 -> Peak CAN Send 0x201/1
  Gain4/1 -> Saturation/1
  Constant2/1 -> Peak CAN Send 0x201/4
  Constant/1 -> Peak CAN Send 0x201/2
  Triggered Subsystem/1(Ready) -> Switch/2
  Constant1/1 -> Switch/1
  Constant3/1 -> Switch/3
  Switch/1 -> Peak CAN Send 0x200/1
  SD-LC Monitor/1(Ready) -> Triggered Subsystem/Trigger
  Constant10/1 -> Peak CAN Send 0x200/7
  Constant9/1 -> Peak CAN Send 0x200/6
  Constant7/1 -> Peak CAN Send 0x200/5
  Constant6/1 -> Peak CAN Send 0x200/4
  Constant5/1 -> Peak CAN Send 0x200/3
  Constant4/1 -> Peak CAN Send 0x200/2

== system Solver_DS_SF/Time Controller ==
  S-Function : S-Function  FunctionName=RT_Enable  Parameters=TimeStep  EnableBusSupport=off
  Terminator : Terminator
  wires:
  S-Function/1 -> Terminator/1

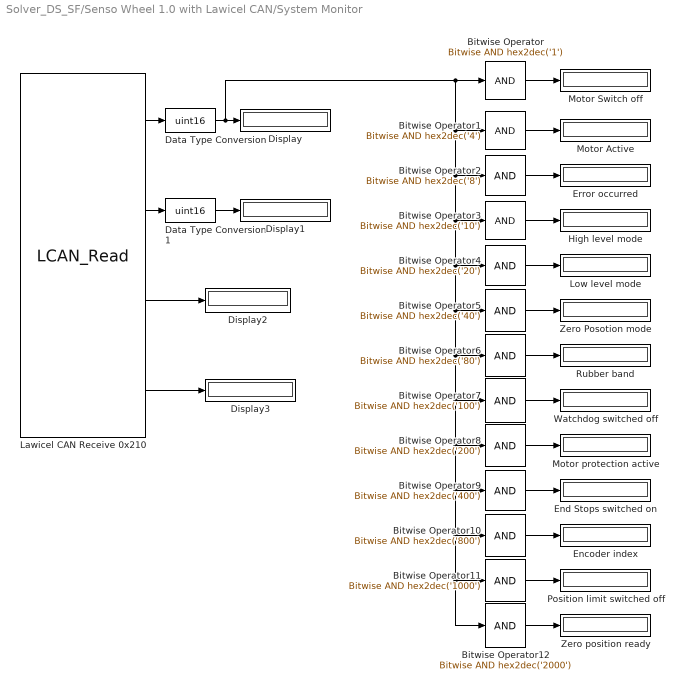
== system Solver_DS_SF/Senso Wheel 1.0 with Lawicel CAN/System Monitor ==
  Bitwise Operator : simulink/Logic and Bit Operations/Bitwise Operator  logicop=AND  UseBitMask=on  BitMask=hex2dec('1')  BitMaskRealWorld=Stored Integer
  Bitwise Operator1 : simulink/Logic and Bit Operations/Bitwise Operator  logicop=AND  UseBitMask=on  BitMask=hex2dec('4')  BitMaskRealWorld=Stored Integer
  Bitwise Operator10 : simulink/Logic and Bit Operations/Bitwise Operator  logicop=AND  UseBitMask=on  BitMask=hex2dec('800')  BitMaskRealWorld=Stored Integer
  Bitwise Operator11 : simulink/Logic and Bit Operations/Bitwise Operator  logicop=AND  UseBitMask=on  BitMask=hex2dec('1000')  BitMaskRealWorld=Stored Integer
  Bitwise Operator12 : simulink/Logic and Bit Operations/Bitwise Operator  logicop=AND  UseBitMask=on  BitMask=hex2dec('2000')  BitMaskRealWorld=Stored Integer
  Bitwise Operator2 : simulink/Logic and Bit Operations/Bitwise Operator  logicop=AND  UseBitMask=on  BitMask=hex2dec('8')  BitMaskRealWorld=Stored Integer
  Bitwise Operator3 : simulink/Logic and Bit Operations/Bitwise Operator  logicop=AND  UseBitMask=on  BitMask=hex2dec('10')  BitMaskRealWorld=Stored Integer
  Bitwise Operator4 : simulink/Logic and Bit Operations/Bitwise Operator  logicop=AND  UseBitMask=on  BitMask=hex2dec('20')  BitMaskRealWorld=Stored Integer
  Bitwise Operator5 : simulink/Logic and Bit Operations/Bitwise Operator  logicop=AND  UseBitMask=on  BitMask=hex2dec('40')  BitMaskRealWorld=Stored Integer
  Bitwise Operator6 : simulink/Logic and Bit Operations/Bitwise Operator  logicop=AND  UseBitMask=on  BitMask=hex2dec('80')  BitMaskRealWorld=Stored Integer
  Bitwise Operator7 : simulink/Logic and Bit Operations/Bitwise Operator  logicop=AND  UseBitMask=on  BitMask=hex2dec('100')  BitMaskRealWorld=Stored Integer
  Bitwise Operator8 : simulink/Logic and Bit Operations/Bitwise Operator  logicop=AND  UseBitMask=on  BitMask=hex2dec('200')  BitMaskRealWorld=Stored Integer
  Bitwise Operator9 : simulink/Logic and Bit Operations/Bitwise Operator  logicop=AND  UseBitMask=on  BitMask=hex2dec('400')  BitMaskRealWorld=Stored Integer
  Data Type Conversion : DataTypeConversion  OutDataTypeStr=uint16  OutDataTypeMode=uint16  RndMeth=Zero
  Data Type Conversion1 : DataTypeConversion  OutDataTypeStr=uint16  OutDataTypeMode=uint16  RndMeth=Zero
  Display{,1..3} (4 alike) : Display
  Encoder index : Display
  End Stops switched on : Display
  Error occurred : Display
  High level mode : Display
  Lawicel CAN Receive 0x210 : S-Function  FunctionName=LCAN_Read  Parameters=1,CAN_MODE,id,TimeStep,nOut,bits_define  EnableBusSupport=off  mask{adapter=CAN1, CAN_MODE=Standard (11-bit), id=528, TimeStep=0.010, bits_define={[0:15],[16:31],[32:47],[48:63]}, portnames={'Status','Errors','End Stop Position','Encodeer Index Position'}}
      mask prompts: adapter "CAN adapter"; CAN_MODE "CAN identifier range:"; id "CAN ID"; TimeStep "Sample time"; bits_define "Bit defination (cell array):"; portnames "Port name (cell array):"
      mask init:
      | nOut=length(bits_define);
      | [bits_define]=formatbit(bits_define,portnames,1);
      | set_param(gcb, 'Parameters', [adapter(4) ',CAN_MODE,id,TimeStep,nOut,bits_define']);
      mask StyleString: popup(CAN1|CAN2|CAN3|CAN4),popup(Standard (11-bit)|Extended (29-bit)),edit,edit,edit,edit
      mask Display: port_label('output',1,'Status ');port_label('output',2,'Errors ');port_label('output',3,'End Stop Position ');port_label('output',4,'Encodeer Index Position ');
  Low level mode : Display
  Motor Active : Display
  Motor Switch off : Display
  Motor protection active : Display
  Position limit switched off : Display
  Rubber band : Display
  Watchdog switched off : Display
  Zero Posotion mode : Display
  Zero position ready : Display
  wires:
  Lawicel CAN Receive 0x210/1 -> Data Type Conversion/1
  Lawicel CAN Receive 0x210/2 -> Data Type Conversion1/1
  Lawicel CAN Receive 0x210/3 -> Display2/1
  Lawicel CAN Receive 0x210/4 -> Display3/1
  Data Type Conversion/1 -> Bitwise Operator/1, Bitwise Operator1/1, Bitwise Operator2/1, Bitwise Operator3/1, Bitwise Operator4/1, Bitwise Operator5/1, Bitwise Operator6/1, Bitwise Operator12/1, Bitwise Operator11/1, Bitwise Operator10/1, Bitwise Operator9/1, Bitwise Operator8/1, Bitwise Operator7/1, Display/1
  Data Type Conversion1/1 -> Display1/1
  Bitwise Operator/1 -> Motor Switch off/1
  Bitwise Operator1/1 -> Motor Active/1
  Bitwise Operator2/1 -> Error occurred/1
  Bitwise Operator3/1 -> High level mode/1
  Bitwise Operator4/1 -> Low level mode/1
  Bitwise Operator5/1 -> Zero Posotion mode/1
  Bitwise Operator6/1 -> Rubber band/1
  Bitwise Operator7/1 -> Watchdog switched off/1
  Bitwise Operator8/1 -> Motor protection active/1
  Bitwise Operator9/1 -> End Stops switched on/1
  Bitwise Operator10/1 -> Encoder index/1
  Bitwise Operator11/1 -> Position limit switched off/1
  Bitwise Operator12/1 -> Zero position ready/1

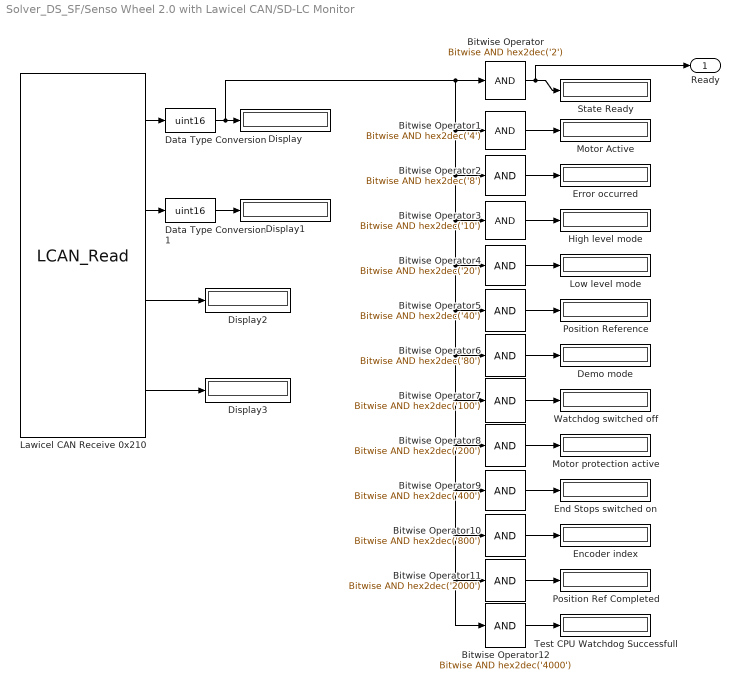
== system Solver_DS_SF/Senso Wheel 2.0 with Lawicel CAN/SD-LC Monitor ==
  Bitwise Operator : simulink/Logic and Bit Operations/Bitwise Operator  logicop=AND  UseBitMask=on  BitMask=hex2dec('2')  BitMaskRealWorld=Stored Integer
  Bitwise Operator1 : simulink/Logic and Bit Operations/Bitwise Operator  logicop=AND  UseBitMask=on  BitMask=hex2dec('4')  BitMaskRealWorld=Stored Integer
  Bitwise Operator10 : simulink/Logic and Bit Operations/Bitwise Operator  logicop=AND  UseBitMask=on  BitMask=hex2dec('800')  BitMaskRealWorld=Stored Integer
  Bitwise Operator11 : simulink/Logic and Bit Operations/Bitwise Operator  logicop=AND  UseBitMask=on  BitMask=hex2dec('2000')  BitMaskRealWorld=Stored Integer
  Bitwise Operator12 : simulink/Logic and Bit Operations/Bitwise Operator  logicop=AND  UseBitMask=on  BitMask=hex2dec('4000')  BitMaskRealWorld=Stored Integer
  Bitwise Operator2 : simulink/Logic and Bit Operations/Bitwise Operator  logicop=AND  UseBitMask=on  BitMask=hex2dec('8')  BitMaskRealWorld=Stored Integer
  Bitwise Operator3 : simulink/Logic and Bit Operations/Bitwise Operator  logicop=AND  UseBitMask=on  BitMask=hex2dec('10')  BitMaskRealWorld=Stored Integer
  Bitwise Operator4 : simulink/Logic and Bit Operations/Bitwise Operator  logicop=AND  UseBitMask=on  BitMask=hex2dec('20')  BitMaskRealWorld=Stored Integer
  Bitwise Operator5 : simulink/Logic and Bit Operations/Bitwise Operator  logicop=AND  UseBitMask=on  BitMask=hex2dec('40')  BitMaskRealWorld=Stored Integer
  Bitwise Operator6 : simulink/Logic and Bit Operations/Bitwise Operator  logicop=AND  UseBitMask=on  BitMask=hex2dec('80')  BitMaskRealWorld=Stored Integer
  Bitwise Operator7 : simulink/Logic and Bit Operations/Bitwise Operator  logicop=AND  UseBitMask=on  BitMask=hex2dec('100')  BitMaskRealWorld=Stored Integer
  Bitwise Operator8 : simulink/Logic and Bit Operations/Bitwise Operator  logicop=AND  UseBitMask=on  BitMask=hex2dec('200')  BitMaskRealWorld=Stored Integer
  Bitwise Operator9 : simulink/Logic and Bit Operations/Bitwise Operator  logicop=AND  UseBitMask=on  BitMask=hex2dec('400')  BitMaskRealWorld=Stored Integer
  Data Type Conversion : DataTypeConversion  OutDataTypeStr=uint16  OutDataTypeMode=uint16  RndMeth=Zero
  Data Type Conversion1 : DataTypeConversion  OutDataTypeStr=uint16  OutDataTypeMode=uint16  RndMeth=Zero
  Demo mode : Display
  Display{,1..3} (4 alike) : Display
  Encoder index : Display
  End Stops switched on : Display
  Error occurred : Display
  High level mode : Display
  Lawicel CAN Receive 0x210 : S-Function  FunctionName=LCAN_Read  Parameters=1,CAN_MODE,id,TimeStep,nOut,bits_define  EnableBusSupport=off  mask{adapter=CAN1, CAN_MODE=Standard (11-bit), id=528, TimeStep=0.1, bits_define={[0:15],[16:31],[32:47],[48:63]}, portnames={'Status','Errors','End Stop Position','Encodeer Index Position'}}
      mask prompts: adapter "CAN adapter"; CAN_MODE "CAN identifier range:"; id "CAN ID"; TimeStep "Sample time"; bits_define "Bit defination (cell array):"; portnames "Port name (cell array):"
      mask init:
      | nOut=length(bits_define);
      | [bits_define]=formatbit(bits_define,portnames,1);
      | set_param(gcb, 'Parameters', [adapter(4) ',CAN_MODE,id,TimeStep,nOut,bits_define']);
      mask StyleString: popup(CAN1|CAN2|CAN3|CAN4),popup(Standard (11-bit)|Extended (29-bit)),edit,edit,edit,edit
      mask Display: port_label('output',1,'Status ');port_label('output',2,'Errors ');port_label('output',3,'End Stop Position ');port_label('output',4,'Encodeer Index Position ');
  Low level mode : Display
  Motor Active : Display
  Motor protection active : Display
  Position Ref Completed : Display
  Position Reference : Display
  State Ready : Display
  Test CPU Watchdog Successfull : Display
  Watchdog switched off : Display
  Ready : Outport  InitialOutput=0
  wires:
  Bitwise Operator12/1 -> Test CPU Watchdog Successfull/1
  Bitwise Operator11/1 -> Position Ref Completed/1
  Bitwise Operator10/1 -> Encoder index/1
  Bitwise Operator9/1 -> End Stops switched on/1
  Bitwise Operator8/1 -> Motor protection active/1
  Bitwise Operator7/1 -> Watchdog switched off/1
  Bitwise Operator6/1 -> Demo mode/1
  Bitwise Operator5/1 -> Position Reference/1
  Bitwise Operator4/1 -> Low level mode/1
  Bitwise Operator3/1 -> High level mode/1
  Bitwise Operator2/1 -> Error occurred/1
  Bitwise Operator1/1 -> Motor Active/1
  Bitwise Operator/1 -> State Ready/1, Ready/1
  Data Type Conversion1/1 -> Display1/1
  Data Type Conversion/1 -> Display/1, Bitwise Operator7/1, Bitwise Operator8/1, Bitwise Operator9/1, Bitwise Operator10/1, Bitwise Operator11/1, Bitwise Operator12/1, Bitwise Operator6/1, Bitwise Operator5/1, Bitwise Operator4/1, Bitwise Operator3/1, Bitwise Operator2/1, Bitwise Operator1/1, Bitwise Operator/1
  Lawicel CAN Receive 0x210/4 -> Display3/1
  Lawicel CAN Receive 0x210/3 -> Display2/1
  Lawicel CAN Receive 0x210/2 -> Data Type Conversion1/1
  Lawicel CAN Receive 0x210/1 -> Data Type Conversion/1

== system Solver_DS_SF/Senso Wheel 2.0 with Lawicel CAN/Triggered Subsystem ==
  Trigger : TriggerPort
  Constant3 : Constant  OutDataTypeStr=uint8  OutDataTypeMode=uint8
  Ready : Outport  InitialOutput=0
  wires:
  Constant3/1 -> Ready/1
